simulink model "Batch_Reactor_Simulation_Series_Reaction2_A_B_C_Approach1"  (R2025a)
settings: Solver=FixedStepAuto  StartTime=0.0  StopTime=50  RelTol=1e-3
settings Model: Creator=must2  LastModifiedBy=must2

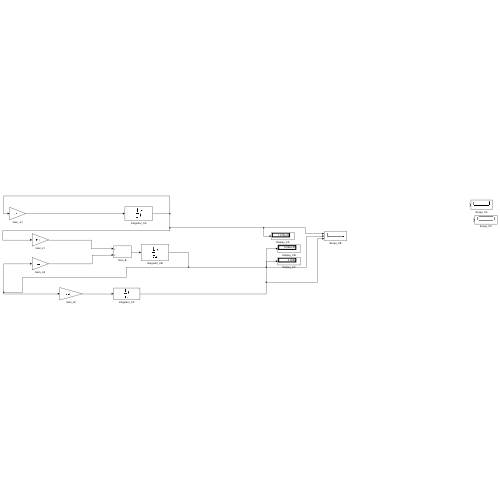
[thumbnail: Simulink's stored preview of the top-level diagram]
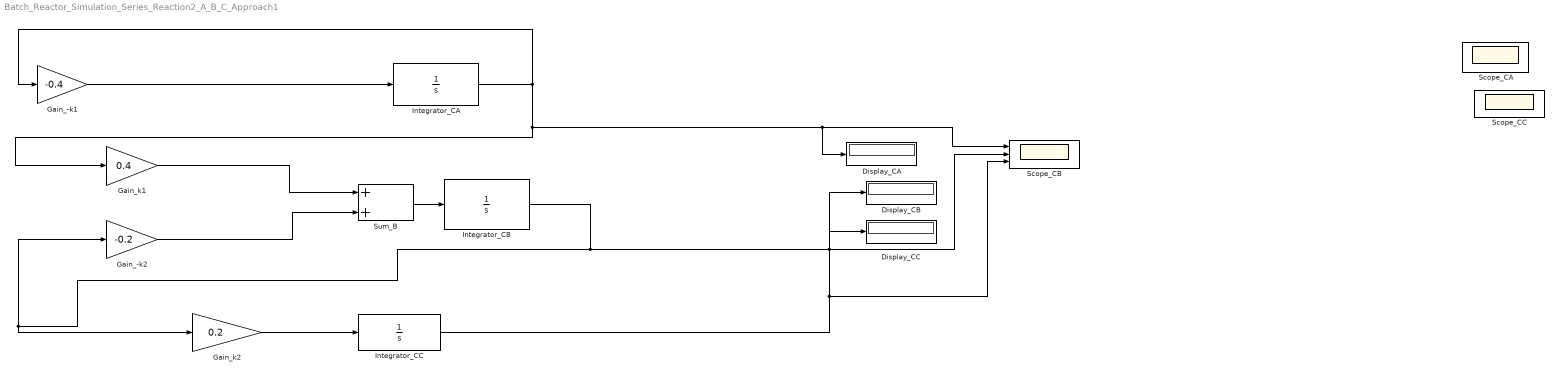
== system Batch_Reactor_Simulation_Series_Reaction2_A_B_C_Approach1 ==
  Display_CA : Display
  Display_CB : Display
  Display_CC : Display
  Gain_-k1 : Gain  Gain=-0.4
  Gain_-k2 : Gain  Gain=-0.2
  Gain_k1 : Gain  Gain=0.4
  Gain_k2 : Gain  Gain=0.2
  Integrator_CA : Integrator  InitialCondition=5  LimitOutput=on  UpperSaturationLimit=1  LowerSaturationLimit=0
  Integrator_CB : Integrator  LimitOutput=on  UpperSaturationLimit=1  LowerSaturationLimit=0
  Integrator_CC : Integrator  LimitOutput=on  UpperSaturationLimit=1  LowerSaturationLimit=0
  Scope_CA : Scope
      settings: ActiveDisplayYMinimum=-0.1249999978458536  ActiveDisplayYMaximum=1.1249999997606503
  Scope_CB : Scope  NumInputPorts=3
      settings: Title=Batch Reactor Simulation: Concentration Profile of A -> B -> C Over Time  ActiveDisplayYMinimum=-0.74861641924614009  ActiveDisplayYMaximum=1.1619994235489424  YLabel=Concentration (mol/L)
  Scope_CC : Scope
      settings: ActiveDisplayYMinimum=-0.1249886945930022  ActiveDisplayYMaximum=1.12489825133702  DataLoggingVariableName=ScopeData2
  Sum_B : Sum
  wires:
  Integrator_CC/1 -> Display_CC/1, Scope_CB/3
  Gain_k1/1 -> Sum_B/1
  Sum_B/1 -> Integrator_CB/1
  Gain_-k2/1 -> Sum_B/2
  Gain_-k1/1 -> Integrator_CA/1
  Gain_k2/1 -> Integrator_CC/1
  Integrator_CA/1 -> Gain_k1/1, Scope_CB/1, Display_CA/1, Gain_-k1/1
  Integrator_CB/1 -> Gain_k2/1, Gain_-k2/1, Scope_CB/2, Display_CB/1
